simulink model "simple_reacher_simulink"  (R2020b)
settings: Solver=VariableStepAuto  StartTime=0.0  StopTime=10.0  RelTol=1e-3
libraries: simulink_gym x2
settings Model: Creator=jbrust  LastModifiedBy=jbrust

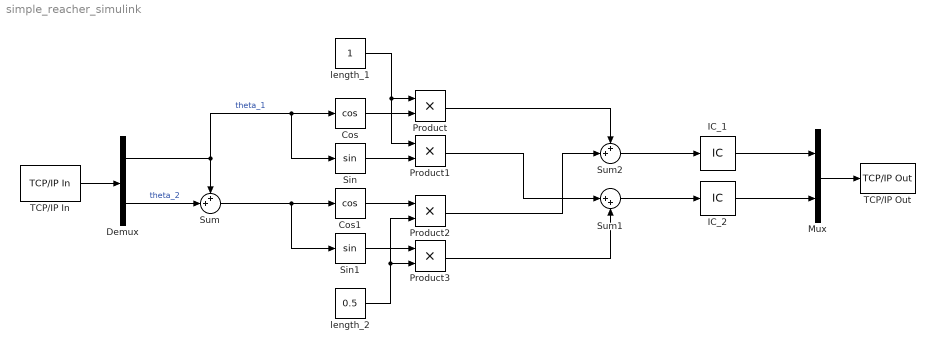
== system simple_reacher_simulink ==
  Cos : Trigonometry  Operator=cos
  Cos1 : Trigonometry  Operator=cos
  Demux : Demux  Outputs=2
  IC_1 : InitialCondition
  IC_2 : InitialCondition
  Mux : Mux  Inputs=2
  Product{,1..3} (4 alike) : Product
  Sin : Trigonometry
  Sin1 : Trigonometry
  Sum : Sum  Inputs=++|
  Sum1 : Sum  Inputs=|++
  Sum2 : Sum  Inputs=++|
  TCP/IP In : simulink_gym/TCP//IP In  Priority=1  port=42313  num_signals=2  t_s=1
      settings: SourceProductName=Simulink Gym
  TCP/IP Out : simulink_gym/TCP//IP Out  Priority=2  port=42312  t_s=1
      settings: SourceProductName=Simulink Gym
  length_1 : Constant
  length_2 : Constant  Value=0.5
  wires:
  TCP/IP In/1 -> Demux/1
  Demux/1 -> Sin/1, Cos/1, Sum/1  "theta_1"
  Sum/1 -> Sin1/1, Cos1/1
  Demux/2 -> Sum/2  "theta_2"
  Mux/1 -> TCP/IP Out/1
  Cos/1 -> Product/2
  length_1/1 -> Product1/1, Product/1
  Sin/1 -> Product1/2
  Sin1/1 -> Product3/1
  Cos1/1 -> Product2/1
  length_2/1 -> Product2/2, Product3/2
  Sum1/1 -> IC_2/1
  Product3/1 -> Sum1/2
  Product1/1 -> Sum1/1
  Sum2/1 -> IC_1/1
  Product/1 -> Sum2/1
  Product2/1 -> Sum2/2
  IC_2/1 -> Mux/2
  IC_1/1 -> Mux/1
